simulink subsystem "Body_Segment_w_Legs"  (R2020b)
settings: Solver=VariableStepAuto  StartTime=0.0  StopTime=10.0  RelTol=1e-3
libraries: nesl_utility x4
settings Model: Creator=theaw  LastModifiedBy=theaw

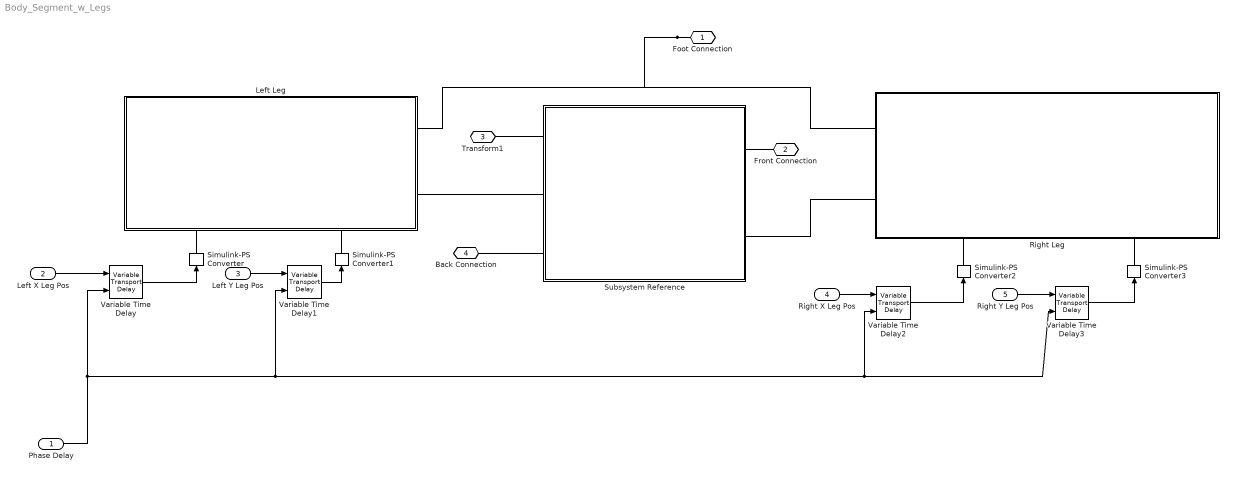
== system Body_Segment_w_Legs ==
  Phase Delay : Inport
  Left X Leg Pos : Inport  Port=2
  Left Y Leg Pos : Inport  Port=3
  Right X Leg Pos : Inport  Port=4
  Right Y Leg Pos : Inport  Port=5
  Left Leg : Subsystem  ReferencedSubsystem=SlideLeg_Simple
      settings: PortSchema="{\"entries\":[{\"content\":{\"sides\":[{\"content\":{\"connectorIds\":[\"LConn4\",\"LConn3\"]},\"type\":\"ConnectorPlacement.EquallySpacedRectSide\",\"uuid\":\"c2ac0ad3-34dd-4924-82c2-819c4b1dda43\"},{\"content\":{\"connectorIds\":[],\"side\":\"RIGHT\"},\"type\":\"ConnectorPlacement.EquallySpacedRectSide\",\"uuid\":\"b434e631-b9e4-407c-a85d-3b43234c48ea\"},{\"content\":{\"connectorIds\":[],\"side\":\"TOP\"},\"type\":\"ConnectorPlacement.EquallySpacedRectSide\",\"uuid\":\"d7aff12c-18af-42f0-8971-b9c4410c2fab\"},{\"content\":{\"connectorIds\":[\"LConn2\",\"LConn1\"],\"side\":\"BOTTOM\"},\"type\":\"ConnectorPlacement.EquallySpacedRectSide\",\"uuid\":\"7d8126e5-56ba-4bc3-a326-8d6189d9accf\"},{\"content\":{\"connectorIds\":[],\"side\":\"HIDDEN\"},\"type\":\"ConnectorPlacement.EquallySpacedRectSide\",\"uuid\":\"dd011aaf-c2d7-4638-9100-c14808993ba5\"}]},\"type\":\"ConnectorPlacement.EquallySpacedConnector\",\"uuid\":\"ccc91101-e749-45fe-97da-50ebed6fec0d\"}],\"packageUris\":[\"http://schema.mathworks.com/mf0/Connector/R2020b\"],\"version\":\"1.0\"}"
  Right Leg : Subsystem  ReferencedSubsystem=SlideLeg_Simple
      settings: PortSchema="{\"entries\":[{\"content\":{\"sides\":[{\"content\":{\"connectorIds\":[\"LConn4\",\"LConn3\"]},\"type\":\"ConnectorPlacement.EquallySpacedRectSide\",\"uuid\":\"c2ac0ad3-34dd-4924-82c2-819c4b1dda43\"},{\"content\":{\"connectorIds\":[],\"side\":\"RIGHT\"},\"type\":\"ConnectorPlacement.EquallySpacedRectSide\",\"uuid\":\"b434e631-b9e4-407c-a85d-3b43234c48ea\"},{\"content\":{\"connectorIds\":[],\"side\":\"TOP\"},\"type\":\"ConnectorPlacement.EquallySpacedRectSide\",\"uuid\":\"d7aff12c-18af-42f0-8971-b9c4410c2fab\"},{\"content\":{\"connectorIds\":[\"LConn1\",\"LConn2\"],\"side\":\"BOTTOM\"},\"type\":\"ConnectorPlacement.EquallySpacedRectSide\",\"uuid\":\"7a89f009-9bc9-48e2-a3d1-97254d4861c7\"},{\"content\":{\"connectorIds\":[],\"side\":\"HIDDEN\"},\"type\":\"ConnectorPlacement.EquallySpacedRectSide\",\"uuid\":\"dd011aaf-c2d7-4638-9100-c14808993ba5\"}]},\"type\":\"ConnectorPlacement.EquallySpacedConnector\",\"uuid\":\"ccc91101-e749-45fe-97da-50ebed6fec0d\"}],\"packageUris\":[\"http://schema.mathworks.com/mf0/Connector/R2020b\"],\"version\":\"1.0\"}"
  Simulink-PS Converter{,1..3} (4 alike) : nesl_utility/Simulink-PS Converter  PhysicalDomain=network_engine_domain  SubClassName=ps_input  LeftPortType=input  RightPortType=output  PseudoPeriodic=off  Frequencies=[]  NoiseDistribution=none  NoiseParameters=[]  Unit=1  AffineConversion=off  FilteringAndDerivatives=filter  SimscapeFilterOrder=2  InputFilterTimeConstant=0.001  UdotUserProvided=0
  Subsystem Reference : Subsystem  ReferencedSubsystem=BodySegment_Rev_Joint
      settings: PortSchema="{\"entries\":[{\"content\":{\"sides\":[{\"content\":{\"connectorIds\":[\"LConn1\",\"LConn3\",\"LConn5\"]},\"type\":\"ConnectorPlacement.EquallySpacedRectSide\",\"uuid\":\"a065fc1c-6e15-4897-9b22-39a911c31a65\"},{\"content\":{\"connectorIds\":[\"LConn4\",\"LConn2\"],\"side\":\"RIGHT\"},\"type\":\"ConnectorPlacement.EquallySpacedRectSide\",\"uuid\":\"4fc3d0ac-d2e5-44fa-94c2-9116087c76bc\"},{\"content\":{\"connectorIds\":[],\"side\":\"TOP\"},\"type\":\"ConnectorPlacement.EquallySpacedRectSide\",\"uuid\":\"806adba4-dd0d-48c9-96a1-fabf5be77dd1\"},{\"content\":{\"connectorIds\":[],\"side\":\"HIDDEN\"},\"type\":\"ConnectorPlacement.EquallySpacedRectSide\",\"uuid\":\"eeecfcc6-42a6-4a57-a7e7-f1b14a64eb77\"}]},\"type\":\"ConnectorPlacement.EquallySpacedConnector\",\"uuid\":\"f05af4c9-8ec1-4ce9-8029-9b20ae18c90c\"}],\"packageUris\":[\"http://schema.mathworks.com/mf0/Connector/R2020b\"],\"version\":\"1.0\"}"
  Variable Time Delay{,1..3} (4 alike) : VariableTransportDelay  MaximumDelay=10
  Foot Connection : PMIOPort  Side=Left
  Front Connection : PMIOPort  Port=2  Side=Left
  Transform1 : PMIOPort  Port=3  Side=Left
  Back Connection : PMIOPort  Port=4  Side=Right
  wires:
  Phase Delay/1 -> Variable Time Delay/2, Variable Time Delay3/2, Variable Time Delay2/2, Variable Time Delay1/2
  Left X Leg Pos/1 -> Variable Time Delay/1
  Variable Time Delay/1 -> Simulink-PS Converter/1
  Variable Time Delay1/1 -> Simulink-PS Converter1/1
  Left Y Leg Pos/1 -> Variable Time Delay1/1
  Right X Leg Pos/1 -> Variable Time Delay2/1
  Variable Time Delay2/1 -> Simulink-PS Converter2/1
  Right Y Leg Pos/1 -> Variable Time Delay3/1
  Variable Time Delay3/1 -> Simulink-PS Converter3/1
  connections:
  Foot Connection/RConn1 -- Left Leg/LConn4 -- Right Leg/LConn4
  Subsystem Reference/LConn4 -- Front Connection/RConn1
  Subsystem Reference/LConn5 -- Back Connection/RConn1
  Subsystem Reference/LConn2 -- Right Leg/LConn3
  Left Leg/LConn3 -- Subsystem Reference/LConn3
  Transform1/RConn1 -- Subsystem Reference/LConn1
  Simulink-PS Converter/RConn1 -- Left Leg/LConn1
  Simulink-PS Converter1/RConn1 -- Left Leg/LConn2
  Simulink-PS Converter2/RConn1 -- Right Leg/LConn1
  Right Leg/LConn2 -- Simulink-PS Converter3/RConn1
